simulink model "All_sensors_Ball_Plate_reduce_observer"  (R2018b)
settings: Solver=ode15s  StartTime=0.0  StopTime=100  RelTol=1e-3
undefined symbols (not defined in the file): A21, B2, Hb, K, K1, K2, K3, K4, X, Y, Z
libraries: sm_lib x16, nesl_utility x11, simulink x3
settings Model: Creator=Giorgio Cannata  LastModifiedBy=Francesca
settings SFSimCC: SimUseLocalCustomCode=off
settings RTWCC: RTWUseLocalCustomCode=off
settings CodeAppCC: StateflowObjectComments=on
settings SimscapeCC: SimscapeNormalizeSystem=off

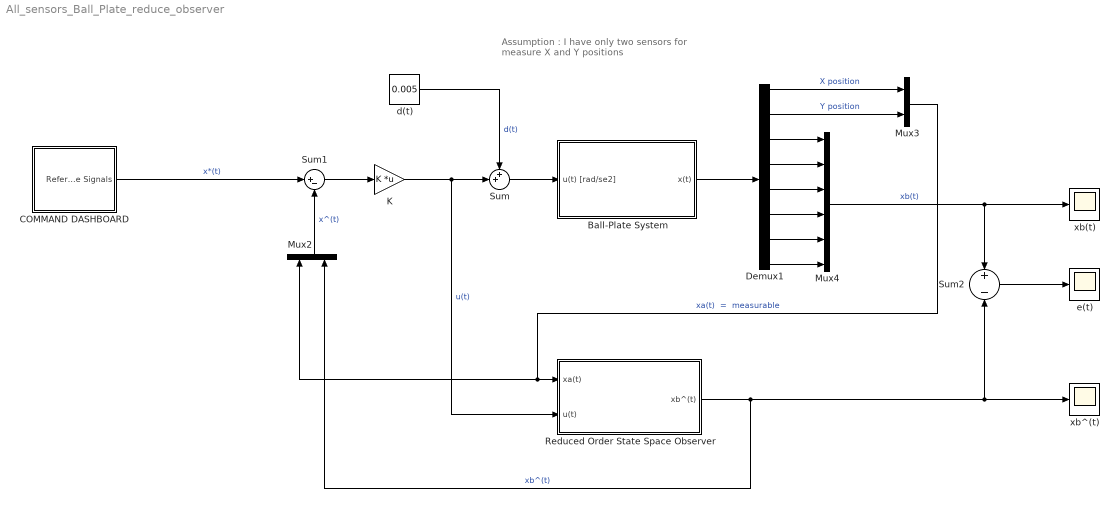
== system All_sensors_Ball_Plate_reduce_observer ==
  note: Assumption : I have only two sensors
      | for measure X and Y positions
  Ball-Plate System : Subsystem  mask{Px0=15, Py0=10, Vx0=0, Vy0=0, alfa0=0, beta0=0, w_alfa0=0, w_beta0=0}
      mask prompts: Px0 "Initial x position [mm]"; Py0 "Initial y position [mm]"; Vx0 "Initial x velocity [mm/sec]"; Vy0 "Initial y velocity [mm/sec]"; alfa0 "Initial alfa angle [deg]"; beta0 "Initial beta angle [deg]"; w_alfa0 "Initial w_alfa [deg/sec]"; w_beta0 "Initial w_beta [deg/sec]"
      mask init:
      | Px0 = Px0/1000;
      | Py0 = Py0/1000;
      | 
      | Vx0 = Vx0/1000;
      | Vy0 = Vy0/1000;
      | 
      | alfa0 = alfa0*pi/180;
      | beta0 = beta0*pi/180;
      | 
      | w_alfa0 = w_alfa0*pi/180;
      | w_beta0 = w_beta0*pi/180;
  COMMAND DASHBOARD : Subsystem
  Demux1 : Demux  Outputs=8
  K : Gain  Gain=K  Multiplication=Matrix(K*u)
  Mux2 : Mux  Inputs=2
  Mux3 : Mux  Inputs=2
  Mux4 : Mux  Inputs=6
  Reduced Order State Space Observer : Subsystem  mask{Hb=Hb, K1=K1, K2=K2, K3=K3, K4=K4}
      mask prompts: Hb "Matrix Hb"; K1 "K1=A22-Hb*A12"; K2 "K2=(A22-Hb*A12)*Hb"; K3 "K3=Hb*B1"; K4 "K4=Hb*A11"
  Sum : Sum  Inputs=++|
  Sum1 : Sum  Inputs=|+-
  Sum2 : Sum  Inputs=+|-
  d(t) : Constant  Value=0.005
  e(t) : Scope
  xb(t) : Scope
  xb^(t) : Scope
  wires:
  COMMAND DASHBOARD/1(Reference Signals) -> Sum1/1  "x*(t)"
  Sum2/1 -> e(t)/1
  K/1 -> Reduced Order State Space Observer/2(u(t)), Sum/2  "u(t)"
  Reduced Order State Space Observer/1(xb^(t)) -> Sum2/2, xb^(t)/1, Mux2/2  "xb^(t)"
  Sum1/1 -> K/1
  d(t)/1 -> Sum/1  "d(t)"
  Sum/1 -> Ball-Plate System/1(u(t) [rad/se2])
  Demux1/7 -> Mux4/5
  Demux1/2 -> Mux3/2  "Y position"
  Demux1/5 -> Mux4/3
  Mux4/1 -> xb(t)/1, Sum2/1  "xb(t)"
  Demux1/8 -> Mux4/6
  Demux1/6 -> Mux4/4
  Ball-Plate System/1(x(t)) -> Demux1/1
  Demux1/1 -> Mux3/1  "X position"
  Demux1/4 -> Mux4/2
  Mux3/1 -> Reduced Order State Space Observer/1(xa(t)), Mux2/1  "xa(t)  =  measurable"
  Demux1/3 -> Mux4/1
  Mux2/1 -> Sum1/2  "x^(t)"

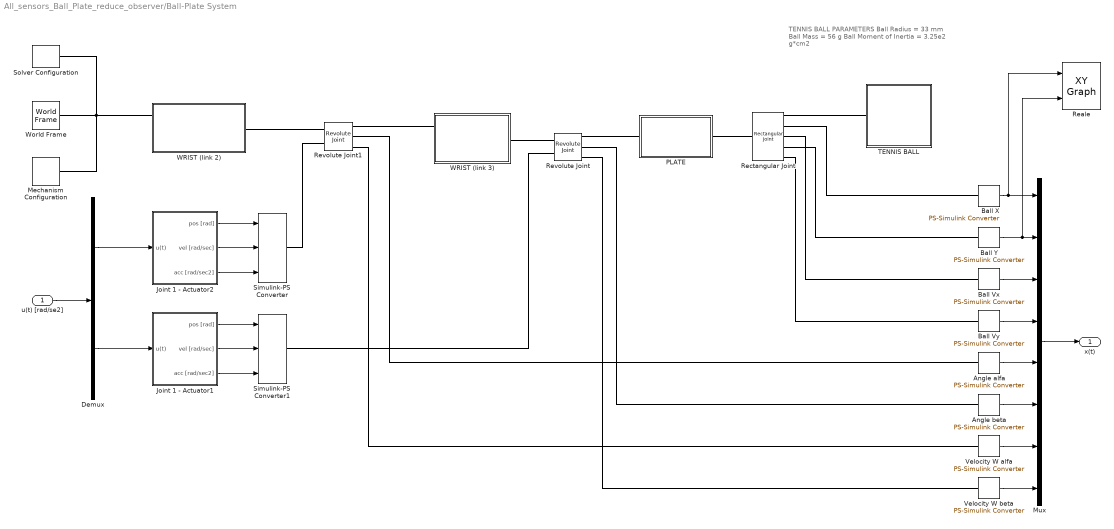
== system All_sensors_Ball_Plate_reduce_observer/Ball-Plate System ==
  note: TENNIS BALL PARAMETERS
      | Ball Radius = 33 mm
      | Ball Mass = 56 g
      | Ball Moment of Inertia = 3.25e2 g*cm2
  u(t) [rad/se2] : Inport
  Angle alfa : nesl_utility/PS-Simulink Converter  PhysicalDomain=network_engine_domain  SubClassName=ps_output  LeftPortType=input  RightPortType=output  PseudoPeriodic=off  Frequencies=[]  Unit=rad  AffineConversion=off
  Angle beta : nesl_utility/PS-Simulink Converter  PhysicalDomain=network_engine_domain  SubClassName=ps_output  LeftPortType=input  RightPortType=output  PseudoPeriodic=off  Frequencies=[]  Unit=rad  AffineConversion=off
  Ball Vx : nesl_utility/PS-Simulink Converter  PhysicalDomain=network_engine_domain  SubClassName=ps_output  LeftPortType=input  RightPortType=output  PseudoPeriodic=off  Frequencies=[]  Unit=m/s  AffineConversion=off
  Ball Vy : nesl_utility/PS-Simulink Converter  PhysicalDomain=network_engine_domain  SubClassName=ps_output  LeftPortType=input  RightPortType=output  PseudoPeriodic=off  Frequencies=[]  Unit=m/s  AffineConversion=off
  Ball X : nesl_utility/PS-Simulink Converter  PhysicalDomain=network_engine_domain  SubClassName=ps_output  LeftPortType=input  RightPortType=output  PseudoPeriodic=off  Frequencies=[]  Unit=m  AffineConversion=off
  Ball Y : nesl_utility/PS-Simulink Converter  PhysicalDomain=network_engine_domain  SubClassName=ps_output  LeftPortType=input  RightPortType=output  PseudoPeriodic=off  Frequencies=[]  Unit=m  AffineConversion=off
  Demux : Demux  Outputs=2
  Joint 1 - Actuator1 : Subsystem  mask{Kp=0, Kv=0, G=1, p0=0, v0=0}
      mask prompts: G "Gain"; p0 "Initial Position [deg]"; v0 "Initial Velocity [deg/sec]"
      mask init:
      | p0 = p0 * pi/180
      | v0 = v0 * pi/180
  Joint 1 - Actuator2 : Subsystem  mask{Kp=0, Kv=0, G=1, p0=0, v0=0}
      mask prompts: G "Gain"; p0 "Initial Position [deg]"; v0 "Initial Velocity [deg/sec]"
      mask init:
      | p0 = p0 * pi/180
      | v0 = v0 * pi/180
  Mechanism Configuration : sm_lib/Utilities/Mechanism Configuration  UniformGravity=Constant  GravityVector=[0 0 -9.80665]  GravityUnits=m/s^2  LinearizationDelta=0.001
  Mux : Mux  Inputs=8
  PLATE : Subsystem  mask{L=400, W=400, T=10, Offset=100}
      mask prompts: L "Plate length [mm]"; W "Plate width [mm]"; T "Plate thickness [mm]"; Offset "Offset [mm]"
  Reale : simulink/Sinks/XY Graph  xmin=-1  xmax=1  ymin=-1  ymax=1  st=-1
  Rectangular Joint : sm_lib/Joints/Rectangular Joint  SenseConstraintForce=off  SenseConstraintForceX=off  SenseConstraintForceY=off  SenseConstraintForceZ=off  SenseConstraintTorque=off  SenseConstraintTorqueX=off  SenseConstraintTorqueY=off  SenseConstraintTorqueZ=off  SenseTotalForce=off  SenseTotalForceX=off  SenseTotalForceY=off  SenseTotalForceZ=off  SenseTotalTorque=off  SenseTotalTorqueX=off  SenseTotalTorqueY=off  SenseTotalTorqueZ=off  CompositeWrenchDir=FollowerOnBase  CompositeWrenchFrame=BaseFrame  PxEquilibriumPosition=0  PxEquilibriumPositionUnits=m  PxSpringStiffness=0  PxSpringStiffnessUnits=N/m  PxDampingCoefficient=0  PxDampingCoefficientUnits=N/(m/s)  PxTorqueActuationMode=NoTorque  PxMotionActuationMode=ComputedMotion  PxSensePosition=on  PxSenseVelocity=on  PxSenseAcceleration=off  PxSenseTorqueForce=off  PxPositionTargetSpecify=on  PxPositionTargetPriority=High  PxPositionTargetValue=Px0  PxPositionTargetValueUnits=m  PxVelocityTargetSpecify=on  PxVelocityTargetPriority=High  PxVelocityTargetValue=Vx0  PxVelocityTargetValueUnits=m/s  PyEquilibriumPosition=0  PyEquilibriumPositionUnits=m  PySpringStiffness=0  PySpringStiffnessUnits=N/m  PyDampingCoefficient=0  PyDampingCoefficientUnits=N/(m/s)  PyTorqueActuationMode=NoTorque  PyMotionActuationMode=ComputedMotion  PySensePosition=on  PySenseVelocity=on  PySenseAcceleration=off  PySenseTorqueForce=off  PyPositionTargetSpecify=on  PyPositionTargetPriority=High  PyPositionTargetValue=Py0  PyPositionTargetValueUnits=m  PyVelocityTargetSpecify=on  PyVelocityTargetPriority=High  PyVelocityTargetValue=Vy0  PyVelocityTargetValueUnits=m/s
      settings: SourceProductName=Simscape Multibody
  Revolute Joint : sm_lib/Joints/Revolute Joint  SenseConstraintForce=off  SenseConstraintForceX=off  SenseConstraintForceY=off  SenseConstraintForceZ=off  SenseConstraintTorque=off  SenseConstraintTorqueX=off  SenseConstraintTorqueY=off  SenseConstraintTorqueZ=off  SenseTotalForce=off  SenseTotalForceX=off  SenseTotalForceY=off  SenseTotalForceZ=off  SenseTotalTorque=off  SenseTotalTorqueX=off  SenseTotalTorqueY=off  SenseTotalTorqueZ=off  CompositeWrenchDir=FollowerOnBase  CompositeWrenchFrame=BaseFrame  EquilibriumPosition=0  EquilibriumPositionUnits=deg  SpringStiffness=0  SpringStiffnessUnits=N*m/deg  DampingCoefficient=0  DampingCoefficientUnits=N*m/(deg/s)  TorqueActuationMode=ComputedTorque  MotionActuationMode=InputMotion  SensePosition=on  SenseVelocity=on  SenseAcceleration=off  SenseTorqueForce=off  PositionTargetSpecify=off  PositionTargetPriority=High  PositionTargetValue=0  PositionTargetValueUnits=deg  VelocityTargetSpecify=off  VelocityTargetPriority=High  VelocityTargetValue=0  VelocityTargetValueUnits=deg/s
  Revolute Joint1 : sm_lib/Joints/Revolute Joint  SenseConstraintForce=off  SenseConstraintForceX=off  SenseConstraintForceY=off  SenseConstraintForceZ=off  SenseConstraintTorque=off  SenseConstraintTorqueX=off  SenseConstraintTorqueY=off  SenseConstraintTorqueZ=off  SenseTotalForce=off  SenseTotalForceX=off  SenseTotalForceY=off  SenseTotalForceZ=off  SenseTotalTorque=off  SenseTotalTorqueX=off  SenseTotalTorqueY=off  SenseTotalTorqueZ=off  CompositeWrenchDir=FollowerOnBase  CompositeWrenchFrame=BaseFrame  EquilibriumPosition=0  EquilibriumPositionUnits=deg  SpringStiffness=0  SpringStiffnessUnits=N*m/deg  DampingCoefficient=0  DampingCoefficientUnits=N*m/(deg/s)  TorqueActuationMode=ComputedTorque  MotionActuationMode=InputMotion  SensePosition=on  SenseVelocity=on  SenseAcceleration=off  SenseTorqueForce=off  PositionTargetSpecify=off  PositionTargetPriority=High  PositionTargetValue=0  PositionTargetValueUnits=deg  VelocityTargetSpecify=off  VelocityTargetPriority=High  VelocityTargetValue=0  VelocityTargetValueUnits=deg/s
  Simulink-PS Converter : nesl_utility/Simulink-PS Converter  PhysicalDomain=network_engine_domain  SubClassName=ps_input  LeftPortType=input  RightPortType=output  PseudoPeriodic=off  Frequencies=[]  NoiseDistribution=none  NoiseParameters=[]  Unit=1  AffineConversion=off  FilteringAndDerivatives=provide  SimscapeFilterOrder=1  InputFilterTimeConstant=0.001  UdotUserProvided=2
  Simulink-PS Converter1 : nesl_utility/Simulink-PS Converter  PhysicalDomain=network_engine_domain  SubClassName=ps_input  LeftPortType=input  RightPortType=output  PseudoPeriodic=off  Frequencies=[]  NoiseDistribution=none  NoiseParameters=[]  Unit=1  AffineConversion=off  FilteringAndDerivatives=provide  SimscapeFilterOrder=1  InputFilterTimeConstant=0.001  UdotUserProvided=2
  Solver Configuration : nesl_utility/Solver Configuration  PhysicalDomain=network_engine_domain  SubClassName=solver  LeftPortType=input  RightPortType=generic  Tones=[]  Harmonics=[]  SimulateNoise=off  Profile=off  UseLocalSampling=off  EnableSwitchedLinearOptims=on  FrequencyDomain=off  UseCCode=off  RelTol=0.001  AbsTol=1e-06  MinStep=1e-09  ToWorkspace=off  RevertToSquareIcSolve=off  NumHomotopyIterations=100  PhasorMode=off  PhasorModeNumHarmonics=1  DoDC=off  ResidualTolerance=1e-09  UseLocalSolver=off  LocalSolverChoice=NE_BACKWARD_EULER_ADVANCER  LocalSolverSampleTime=0.0005  DoFixedCost=off  MaxNonlinIter=3  MaxModeIter=2  LinearAlgebra=Sparse  EquationFormulation=NE_TIME_EF  DelaysMemoryBudget=1024  AutomaticFiltering=on  FilteringTimeConstant=0.001  PartitionStorageMethod=AS_NEEDED  PartitionMemoryBudget=1024
  TENNIS BALL : Subsystem  mask{rb=33, mb=56, Ib=3.25e2}
      mask prompts: rb "Ball radius [mm]"; mb "Ball mass [g]"; Ib "Ball momentum of inertia [g cm2]"
      mask init:
      | Ib = 10^4 * Ib; % Trasnfor to [g*mm]
      | m = mb + Ib/rb^2; % Equivalent inertia - as a sliding object
      mask Display: image('TennisBall.png');
  Velocity W alfa : nesl_utility/PS-Simulink Converter  PhysicalDomain=network_engine_domain  SubClassName=ps_output  LeftPortType=input  RightPortType=output  PseudoPeriodic=off  Frequencies=[]  Unit=rad/s  AffineConversion=off
  Velocity W beta : nesl_utility/PS-Simulink Converter  PhysicalDomain=network_engine_domain  SubClassName=ps_output  LeftPortType=input  RightPortType=output  PseudoPeriodic=off  Frequencies=[]  Unit=rad/s  AffineConversion=off
  WRIST (link 2) : Subsystem  mask{L=150, R=80}
      mask prompts: L "Length [mm]"; R "Radius [mm]"
  WRIST (link 3) : Subsystem  mask{L=300, R=65}
      mask prompts: L "Link length [mm]"; R "Link radius [mm]"
  World Frame : sm_lib/Frames and Transforms/World Frame
  x(t) : Outport
  wires:
  Angle alfa/1 -> Mux/5
  Ball Vy/1 -> Mux/4
  Angle beta/1 -> Mux/6
  Ball Vx/1 -> Mux/3
  Ball Y/1 -> Reale/2, Mux/2
  Velocity W alfa/1 -> Mux/7
  Ball X/1 -> Mux/1, Reale/1
  Velocity W beta/1 -> Mux/8
  u(t) [rad/se2]/1 -> Demux/1
  Mux/1 -> x(t)/1
  Demux/1 -> Joint 1 - Actuator2/1(u(t))
  Joint 1 - Actuator2/1(pos [rad]) -> Simulink-PS Converter/1
  Joint 1 - Actuator2/2(vel [rad/sec]) -> Simulink-PS Converter/2
  Joint 1 - Actuator2/3(acc [rad/sec2]) -> Simulink-PS Converter/3
  Joint 1 - Actuator1/1(pos [rad]) -> Simulink-PS Converter1/1
  Joint 1 - Actuator1/2(vel [rad/sec]) -> Simulink-PS Converter1/2
  Joint 1 - Actuator1/3(acc [rad/sec2]) -> Simulink-PS Converter1/3
  Demux/2 -> Joint 1 - Actuator1/1(u(t))
  connections:
  WRIST (link 3)/RConn1 -- Revolute Joint/LConn1
  Revolute Joint1/LConn1 -- WRIST (link 2)/RConn1
  Revolute Joint/RConn1 -- PLATE/LConn1
  PLATE/RConn1 -- Rectangular Joint/LConn1
  TENNIS BALL/LConn1 -- Rectangular Joint/RConn1
  Ball X/LConn1 -- Rectangular Joint/RConn2
  Revolute Joint1/RConn1 -- WRIST (link 3)/LConn1
  Solver Configuration/RConn1 -- WRIST (link 2)/LConn1 -- Mechanism Configuration/RConn1 -- World Frame/RConn1
  Rectangular Joint/RConn4 -- Ball Y/LConn1
  Rectangular Joint/RConn3 -- Ball Vx/LConn1
  Rectangular Joint/RConn5 -- Ball Vy/LConn1
  Revolute Joint/RConn2 -- Angle beta/LConn1
  Revolute Joint1/RConn2 -- Angle alfa/LConn1
  Revolute Joint1/RConn3 -- Velocity W alfa/LConn1
  Revolute Joint/RConn3 -- Velocity W beta/LConn1
  Simulink-PS Converter/RConn1 -- Revolute Joint1/LConn2
  Simulink-PS Converter1/RConn1 -- Revolute Joint/LConn2

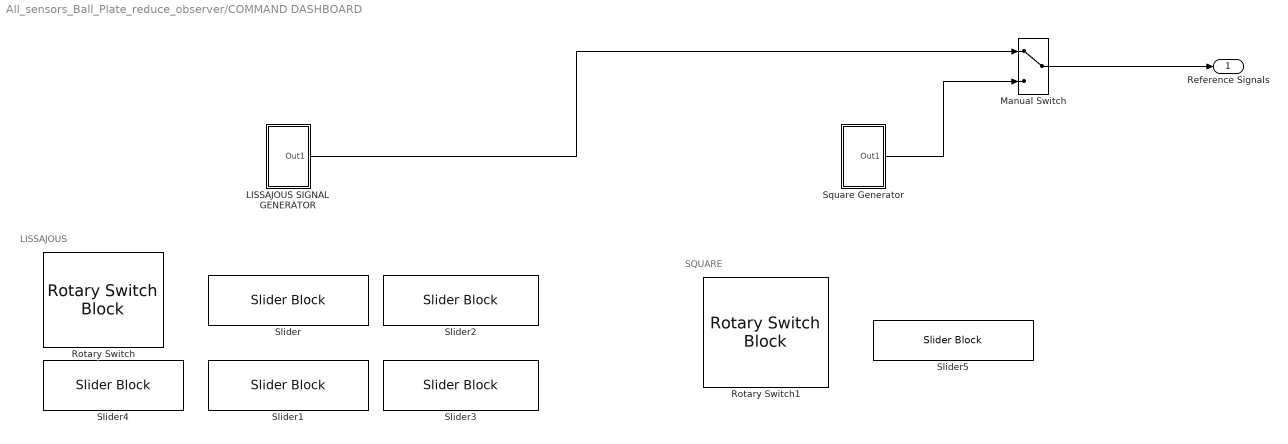
== system All_sensors_Ball_Plate_reduce_observer/COMMAND DASHBOARD ==
  note: SQUARE
  note: LISSAJOUS
  LISSAJOUS SIGNAL GENERATOR : Subsystem
  Manual Switch : ManualSwitch
  Rotary Switch : RotarySwitchBlock  WebBlockId=121
      settings: Values={{'X-Y', 'L (1-1)', 'L (1-2)', 'L (3-2)', 'L (3-4)', 'L (5-4)'}, [0 1 2 3 4 5]}
  Rotary Switch1 : RotarySwitchBlock  WebBlockId=120
      settings: Values={{'Low', 'Low-Med', 'Med-High', 'High', 'Very-High'}, [3 5 7 9 11]}
  Slider : SliderBlock  WebBlockId=119  ScaleMax=0.20000000000000001
  Slider1 : SliderBlock  WebBlockId=118  ScaleMax=0.20000000000000001
  Slider2 : SliderBlock  WebBlockId=117  ScaleMin=-0.20000000000000001  ScaleMax=0.20000000000000001
  Slider3 : SliderBlock  WebBlockId=115  ScaleMin=-0.20000000000000001  ScaleMax=0.20000000000000001
  Slider4 : SliderBlock  WebBlockId=116  ScaleMax=1
  Slider5 : SliderBlock  WebBlockId=114  ScaleMax=2
  Square Generator : Subsystem
  Reference Signals : Outport
  wires:
  Square Generator/1(Out1) -> Manual Switch/2
  Manual Switch/1 -> Reference Signals/1
  LISSAJOUS SIGNAL GENERATOR/1(Out1) -> Manual Switch/1

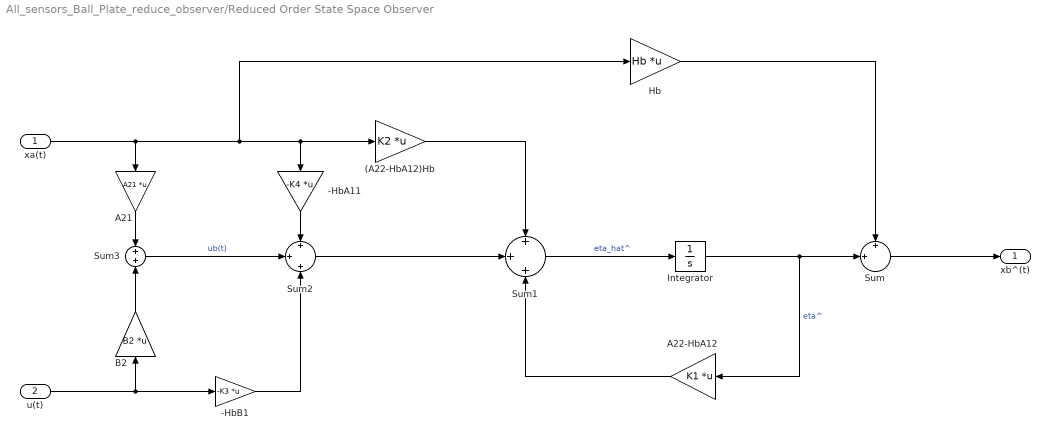
== system All_sensors_Ball_Plate_reduce_observer/Reduced Order State Space Observer ==
  xa(t) : Inport
  u(t) : Inport  Port=2
  (A22-HbA12)Hb : Gain  Gain=K2  Multiplication=Matrix(K*u)
  -HbA11 : Gain  Gain=-K4  Multiplication=Matrix(K*u)
  -HbB1 : Gain  Gain=-K3  Multiplication=Matrix(K*u)
  A21 : Gain  Gain=A21  Multiplication=Matrix(K*u)
  A22-HbA12 : Gain  Gain=K1  Multiplication=Matrix(K*u)
  B2 : Gain  Gain=B2  Multiplication=Matrix(K*u)
  Hb : Gain  Gain=Hb  Multiplication=Matrix(K*u)
  Integrator : Integrator
  Sum : Sum  Inputs=+|+||
  Sum1 : Sum  Inputs=+|+|+
  Sum2 : Sum  Inputs=+|+|+
  Sum3 : Sum  Inputs=+|+
  xb^(t) : Outport
  wires:
  Hb/1 -> Sum/1
  A21/1 -> Sum3/1
  (A22-HbA12)Hb/1 -> Sum1/1
  B2/1 -> Sum3/2
  A22-HbA12/1 -> Sum1/3
  u(t)/1 -> -HbB1/1, B2/1
  Sum1/1 -> Integrator/1  "eta_hat^"
  -HbA11/1 -> Sum2/1
  Sum2/1 -> Sum1/2
  Sum/1 -> xb^(t)/1
  Integrator/1 -> Sum/2, A22-HbA12/1  "eta^"
  xa(t)/1 -> Hb/1, -HbA11/1, (A22-HbA12)Hb/1, A21/1
  Sum3/1 -> Sum2/2  "ub(t)"
  -HbB1/1 -> Sum2/3

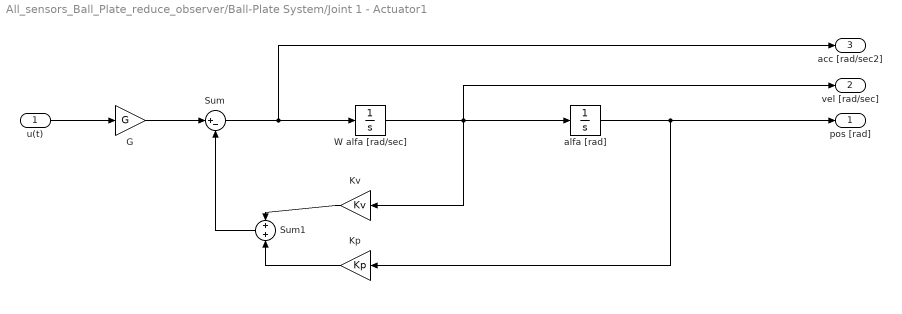
== system All_sensors_Ball_Plate_reduce_observer/Ball-Plate System/Joint 1 - Actuator1 ==
  u(t) : Inport
  G : Gain  Gain=G
  Kp : Gain  Gain=Kp
  Kv : Gain  Gain=Kv
  Sum : Sum  Inputs=|+-
  Sum1 : Sum  Inputs=+|+
  W alfa [rad/sec] : Integrator  InitialCondition=v0
  alfa [rad] : Integrator  InitialCondition=p0
  pos [rad] : Outport
  vel [rad/sec] : Outport  Port=2
  acc [rad/sec2] : Outport  Port=3
  wires:
  Sum1/1 -> Sum/2
  Kp/1 -> Sum1/2
  Kv/1 -> Sum1/1
  G/1 -> Sum/1
  Sum/1 -> W alfa [rad/sec]/1, acc [rad/sec2]/1
  alfa [rad]/1 -> pos [rad]/1, Kp/1
  W alfa [rad/sec]/1 -> alfa [rad]/1, vel [rad/sec]/1, Kv/1
  u(t)/1 -> G/1

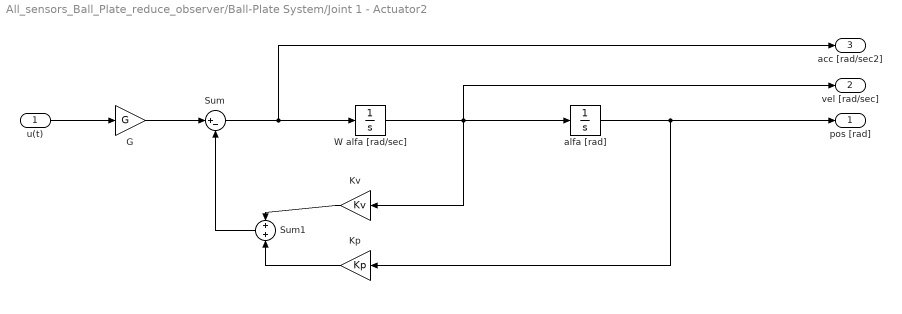
== system All_sensors_Ball_Plate_reduce_observer/Ball-Plate System/Joint 1 - Actuator2 ==
  u(t) : Inport
  G : Gain  Gain=G
  Kp : Gain  Gain=Kp
  Kv : Gain  Gain=Kv
  Sum : Sum  Inputs=|+-
  Sum1 : Sum  Inputs=+|+
  W alfa [rad/sec] : Integrator  InitialCondition=v0
  alfa [rad] : Integrator  InitialCondition=p0
  pos [rad] : Outport
  vel [rad/sec] : Outport  Port=2
  acc [rad/sec2] : Outport  Port=3
  wires:
  u(t)/1 -> G/1
  W alfa [rad/sec]/1 -> Kv/1, vel [rad/sec]/1, alfa [rad]/1
  alfa [rad]/1 -> Kp/1, pos [rad]/1
  Sum/1 -> acc [rad/sec2]/1, W alfa [rad/sec]/1
  G/1 -> Sum/1
  Kv/1 -> Sum1/1
  Kp/1 -> Sum1/2
  Sum1/1 -> Sum/2

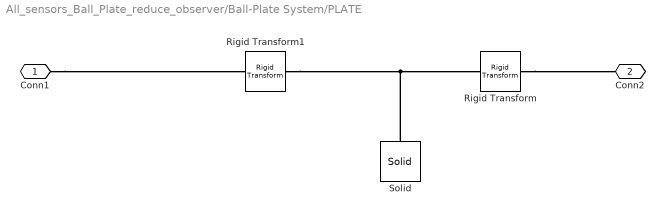
== system All_sensors_Ball_Plate_reduce_observer/Ball-Plate System/PLATE ==
  Rigid Transform : sm_lib/Frames and Transforms/Rigid Transform  TranslationMethod=StandardAxis  TranslationStandardOffset=T/2  TranslationLengthUnit=mm  TranslationStandardAxis=+Z  TranslationCartesianOffset=[0 0 0]  TranslationROffset=0  TranslationROffsetUnits=m  TranslationZOffset=0  TranslationZOffsetUnits=m  TranslationThetaOffset=0  TranslationThetaOffsetUnits=deg  RotationMethod=None  RotationAngleUnits=deg  RotationStandardAxis=+Z  RotationAngle=0.0  RotationArbitraryAxis=[0 0 1]  FollAlignAxisA=+X  BaseAlignAxisA=+Y  FollAlignAxisB=+Y  BaseAlignAxisB=+Z  RotationSequenceAxes=FollowerAxes  RotationSequence=XYX  RotationSequenceAngles=[0 0 0]  RotationSequenceAnglesUnits=deg  RotationMatrix=[1 0 0; 0 1 0; 0 0 1]
  Rigid Transform1 : sm_lib/Frames and Transforms/Rigid Transform  TranslationMethod=StandardAxis  TranslationStandardOffset=Offset-T/2  TranslationLengthUnit=mm  TranslationStandardAxis=-Z  TranslationCartesianOffset=[0 0 0]  TranslationROffset=0  TranslationROffsetUnits=m  TranslationZOffset=0  TranslationZOffsetUnits=m  TranslationThetaOffset=0  TranslationThetaOffsetUnits=deg  RotationMethod=StandardAxis  RotationAngleUnits=deg  RotationStandardAxis=-X  RotationAngle=90.0  RotationArbitraryAxis=[1 0 0]  FollAlignAxisA=+X  BaseAlignAxisA=+Y  FollAlignAxisB=+Y  BaseAlignAxisB=+Z  RotationSequenceAxes=FollowerAxes  RotationSequence=XYX  RotationSequenceAngles=[0 0 0]  RotationSequenceAnglesUnits=deg  RotationMatrix=[1 0 0; 0 1 0; 0 0 1]
  Solid : sm_lib/Body Elements/Solid  InertiaType=CalculateFromGeometry  Mass=1  MassUnits=kg  CenterOfMass=[0 0 0]  CenterOfMassUnits=m  MomentsOfInertia=[1 1 1]  MomentsOfInertiaUnits=kg*m^2  ProductsOfInertia=[0 0 0]  ProductsOfInertiaUnits=kg*m^2  BasedOnType=Density  Density=0  DensityUnits=kg/(m^3)  DoExposeReferenceFrame=on  SerializedFrames=<Frames/>  GraphicType=FromGeometry  MarkerShape=Sphere  MarkerSize=10  GraphicVisPropType=SimpleVisualProperties  GraphicDiffuseColor=[0.65 0.65 0.65]  GraphicSpecularColor=[0.5 0.5 0.5 1.0]  GraphicAmbientColor=[0.15 0.15 0.15 1.0]  GraphicEmissiveColor=[0.0 0.0 0.0 1.0]  GraphicShininess=75  GraphicOpacity=1.0  GeometryShape=Brick  RectangleSize=[1 1]  RectangleSizeUnits=m  BrickDimensions=[L W T]  BrickDimensionUnits=mm  CylinderRadius=1  CylinderRadiusUnits=m  CylinderLength=1  CylinderLengthUnits=m  SphereRadius=1  SphereRadiusUnits=m  EllipsoidRadii=[1 1 1]  EllipsoidRadiiUnits=m  ExtrusionCrossSection=[1 1; -1 1; -1 -1; 1 -1]  ExtrusionCrossSectionUnits=m  ExtrusionLength=1  ExtrusionLengthUnits=m  PolygonNumSides=3  PolygonOuterRadius=1  PolygonOuterRadiusUnits=m  ExtGeomFileType=STEP  ExtGeomFileUnits=m  RevolutionCrossSection=[1 1; 1 -1; 2 -1; 2 1]  RevolutionCrossSectionUnits=m  RevolutionExtent=Full  RevolutionAngle=180  RevolutionAngleUnits=deg
  Conn1 : PMIOPort  Side=Left
  Conn2 : PMIOPort  Port=2  Side=Right
  connections:
  Rigid Transform/RConn1 -- Conn2/RConn1
  Conn1/RConn1 -- Rigid Transform1/RConn1
  Rigid Transform1/LConn1 -- Solid/RConn1 -- Rigid Transform/LConn1

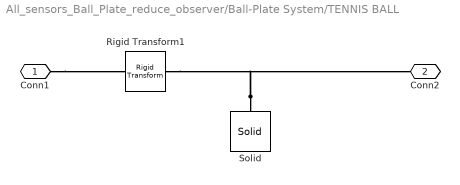
== system All_sensors_Ball_Plate_reduce_observer/Ball-Plate System/TENNIS BALL ==
  Rigid Transform1 : sm_lib/Frames and Transforms/Rigid Transform  TranslationMethod=StandardAxis  TranslationStandardOffset=rb  TranslationLengthUnit=mm  TranslationStandardAxis=-Z  TranslationCartesianOffset=[0 0 0]  TranslationROffset=0  TranslationROffsetUnits=m  TranslationZOffset=0  TranslationZOffsetUnits=m  TranslationThetaOffset=0  TranslationThetaOffsetUnits=deg  RotationMethod=None  RotationAngleUnits=deg  RotationStandardAxis=+Z  RotationAngle=0.0  RotationArbitraryAxis=[0 0 1]  FollAlignAxisA=+X  BaseAlignAxisA=+Y  FollAlignAxisB=+Y  BaseAlignAxisB=+Z  RotationSequenceAxes=FollowerAxes  RotationSequence=XYX  RotationSequenceAngles=[0 0 0]  RotationSequenceAnglesUnits=deg  RotationMatrix=[1 0 0; 0 1 0; 0 0 1]
  Solid : sm_lib/Body Elements/Solid  InertiaType=Custom  Mass=m  MassUnits=g  CenterOfMass=[0 0 0]  CenterOfMassUnits=mm  MomentsOfInertia=[1 1 1]*0  MomentsOfInertiaUnits=g*cm^2  ProductsOfInertia=[0 0 0]  ProductsOfInertiaUnits=kg*m^2  BasedOnType=Density  Density=1000  DensityUnits=kg/(m^3)  DoExposeReferenceFrame=on  SerializedFrames=<Frames/>  GraphicType=FromGeometry  MarkerShape=Sphere  MarkerSize=10  GraphicVisPropType=AdvancedVisualProperties  GraphicDiffuseColor=[1 1 0]  GraphicSpecularColor=[1 1 0 1]  GraphicAmbientColor=[0.15 0.15 0.15 1.0]  GraphicEmissiveColor=[0.1 0.1 0.0 1.0]  GraphicShininess=10  GraphicOpacity=1.0  GeometryShape=Sphere  RectangleSize=[1 1]  RectangleSizeUnits=m  BrickDimensions=[1 1 1]  BrickDimensionUnits=m  CylinderRadius=1  CylinderRadiusUnits=m  CylinderLength=1  CylinderLengthUnits=m  SphereRadius=rb  SphereRadiusUnits=mm  EllipsoidRadii=[1 1 1]  EllipsoidRadiiUnits=m  ExtrusionCrossSection=[1 1; -1 1; -1 -1; 1 -1]  ExtrusionCrossSectionUnits=m  ExtrusionLength=1  ExtrusionLengthUnits=m  PolygonNumSides=3  PolygonOuterRadius=1  PolygonOuterRadiusUnits=m  ExtGeomFileType=STEP  ExtGeomFileUnits=m  RevolutionCrossSection=[1 1; 1 -1; 2 -1; 2 1]  RevolutionCrossSectionUnits=m  RevolutionExtent=Full  RevolutionAngle=180  RevolutionAngleUnits=deg
  Conn1 : PMIOPort  Side=Left
  Conn2 : PMIOPort  Port=2  Side=Right
  connections:
  Conn1/RConn1 -- Rigid Transform1/RConn1
  Solid/RConn1 -- Rigid Transform1/LConn1 -- Conn2/RConn1

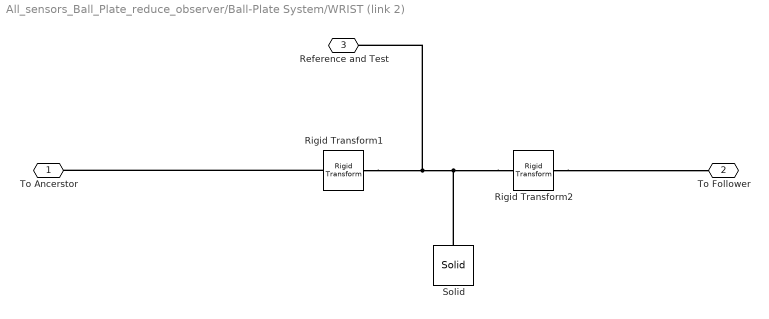
== system All_sensors_Ball_Plate_reduce_observer/Ball-Plate System/WRIST (link 2) ==
  Rigid Transform1 : sm_lib/Frames and Transforms/Rigid Transform  TranslationMethod=None  TranslationStandardOffset=L/2  TranslationLengthUnit=mm  TranslationStandardAxis=-Z  TranslationCartesianOffset=[0 0 0]  TranslationROffset=0  TranslationROffsetUnits=m  TranslationZOffset=0  TranslationZOffsetUnits=m  TranslationThetaOffset=0  TranslationThetaOffsetUnits=deg  RotationMethod=StandardAxis  RotationAngleUnits=deg  RotationStandardAxis=+Y  RotationAngle=-90.0  RotationArbitraryAxis=[1 0 0]  FollAlignAxisA=+X  BaseAlignAxisA=+Y  FollAlignAxisB=+Y  BaseAlignAxisB=+Z  RotationSequenceAxes=FollowerAxes  RotationSequence=XYX  RotationSequenceAngles=[0 0 0]  RotationSequenceAnglesUnits=deg  RotationMatrix=[1 0 0; 0 1 0; 0 0 1]
  Rigid Transform2 : sm_lib/Frames and Transforms/Rigid Transform  TranslationMethod=None  TranslationStandardOffset=L/2  TranslationLengthUnit=mm  TranslationStandardAxis=+Z  TranslationCartesianOffset=[0 0 0]  TranslationROffset=0  TranslationROffsetUnits=m  TranslationZOffset=0  TranslationZOffsetUnits=m  TranslationThetaOffset=0  TranslationThetaOffsetUnits=deg  RotationMethod=None  RotationAngleUnits=deg  RotationStandardAxis=+Z  RotationAngle=-90.0  RotationArbitraryAxis=[1 0 0]  FollAlignAxisA=+X  BaseAlignAxisA=+Y  FollAlignAxisB=+Y  BaseAlignAxisB=+Z  RotationSequenceAxes=FollowerAxes  RotationSequence=XYX  RotationSequenceAngles=[0 0 0]  RotationSequenceAnglesUnits=deg  RotationMatrix=[1 0 0; 0 1 0; 0 0 1]
  Solid : sm_lib/Body Elements/Solid  InertiaType=CalculateFromGeometry  Mass=1  MassUnits=kg  CenterOfMass=[0 0 0]  CenterOfMassUnits=m  MomentsOfInertia=[1 1 1]  MomentsOfInertiaUnits=kg*m^2  ProductsOfInertia=[0 0 0]  ProductsOfInertiaUnits=kg*m^2  BasedOnType=Density  Density=0  DensityUnits=kg/(m^3)  DoExposeReferenceFrame=on  SerializedFrames=<Frames/>  GraphicType=FromGeometry  MarkerShape=Sphere  MarkerSize=10  GraphicVisPropType=SimpleVisualProperties  GraphicDiffuseColor=[0.65 00.15 0.35]  GraphicSpecularColor=[0.5 0.5 0.5 1.0]  GraphicAmbientColor=[0.15 0.15 0.15 1.0]  GraphicEmissiveColor=[0.0 0.0 0.0 1.0]  GraphicShininess=75  GraphicOpacity=1.0  GeometryShape=Cylinder  RectangleSize=[1 1]  RectangleSizeUnits=m  BrickDimensions=[1 1 1]  BrickDimensionUnits=m  CylinderRadius=R  CylinderRadiusUnits=mm  CylinderLength=L  CylinderLengthUnits=mm  SphereRadius=1  SphereRadiusUnits=m  EllipsoidRadii=[1 1 1]  EllipsoidRadiiUnits=m  ExtrusionCrossSection=[1 1; -1 1; -1 -1; 1 -1]  ExtrusionCrossSectionUnits=m  ExtrusionLength=1  ExtrusionLengthUnits=m  PolygonNumSides=3  PolygonOuterRadius=1  PolygonOuterRadiusUnits=m  ExtGeomFileType=STEP  ExtGeomFileUnits=m  RevolutionCrossSection=[1 1; 1 -1; 2 -1; 2 1]  RevolutionCrossSectionUnits=m  RevolutionExtent=Full  RevolutionAngle=180  RevolutionAngleUnits=deg
  To Ancerstor : PMIOPort  Side=Left
  To Follower : PMIOPort  Port=2  Side=Right
  Reference and Test : PMIOPort  Port=3  Side=Left
  connections:
  Rigid Transform2/LConn1 -- Reference and Test/RConn1 -- Rigid Transform1/LConn1 -- Solid/RConn1
  Rigid Transform1/RConn1 -- To Ancerstor/RConn1
  Rigid Transform2/RConn1 -- To Follower/RConn1

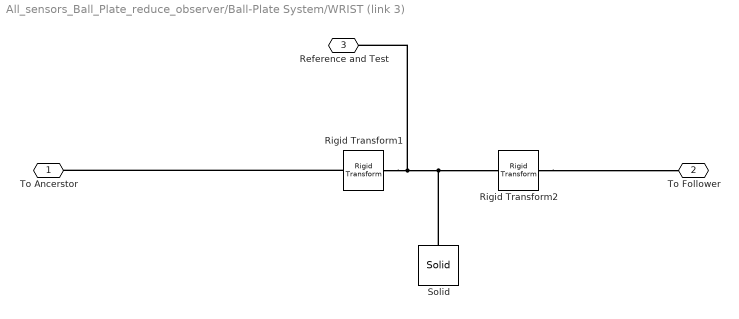
== system All_sensors_Ball_Plate_reduce_observer/Ball-Plate System/WRIST (link 3) ==
  Rigid Transform1 : sm_lib/Frames and Transforms/Rigid Transform  TranslationMethod=StandardAxis  TranslationStandardOffset=L/2  TranslationLengthUnit=mm  TranslationStandardAxis=-Z  TranslationCartesianOffset=[0 0 0]  TranslationROffset=0  TranslationROffsetUnits=m  TranslationZOffset=0  TranslationZOffsetUnits=m  TranslationThetaOffset=0  TranslationThetaOffsetUnits=deg  RotationMethod=StandardAxis  RotationAngleUnits=deg  RotationStandardAxis=+X  RotationAngle=90.0  RotationArbitraryAxis=[1 0 0]  FollAlignAxisA=+X  BaseAlignAxisA=+Y  FollAlignAxisB=+Y  BaseAlignAxisB=+Z  RotationSequenceAxes=FollowerAxes  RotationSequence=XYX  RotationSequenceAngles=[0 0 0]  RotationSequenceAnglesUnits=deg  RotationMatrix=[1 0 0; 0 1 0; 0 0 1]
  Rigid Transform2 : sm_lib/Frames and Transforms/Rigid Transform  TranslationMethod=StandardAxis  TranslationStandardOffset=L/2  TranslationLengthUnit=mm  TranslationStandardAxis=+Z  TranslationCartesianOffset=[0 0 0]  TranslationROffset=0  TranslationROffsetUnits=m  TranslationZOffset=0  TranslationZOffsetUnits=m  TranslationThetaOffset=0  TranslationThetaOffsetUnits=deg  RotationMethod=StandardAxis  RotationAngleUnits=deg  RotationStandardAxis=+Z  RotationAngle=-90.0  RotationArbitraryAxis=[1 0 0]  FollAlignAxisA=+X  BaseAlignAxisA=+Y  FollAlignAxisB=+Y  BaseAlignAxisB=+Z  RotationSequenceAxes=FollowerAxes  RotationSequence=XYX  RotationSequenceAngles=[0 0 0]  RotationSequenceAnglesUnits=deg  RotationMatrix=[1 0 0; 0 1 0; 0 0 1]
  Solid : sm_lib/Body Elements/Solid  InertiaType=CalculateFromGeometry  Mass=1  MassUnits=kg  CenterOfMass=[0 0 0]  CenterOfMassUnits=m  MomentsOfInertia=[1 1 1]  MomentsOfInertiaUnits=kg*m^2  ProductsOfInertia=[0 0 0]  ProductsOfInertiaUnits=kg*m^2  BasedOnType=Density  Density=0  DensityUnits=kg/(m^3)  DoExposeReferenceFrame=on  SerializedFrames=<Frames/>  GraphicType=FromGeometry  MarkerShape=Sphere  MarkerSize=10  GraphicVisPropType=SimpleVisualProperties  GraphicDiffuseColor=[0.65 0 0]  GraphicSpecularColor=[0.5 0.5 0.5 1.0]  GraphicAmbientColor=[0.15 0.15 0.15 1.0]  GraphicEmissiveColor=[0.0 0.0 0.0 1.0]  GraphicShininess=75  GraphicOpacity=1.0  GeometryShape=Cylinder  RectangleSize=[1 1]  RectangleSizeUnits=m  BrickDimensions=[1 1 1]  BrickDimensionUnits=m  CylinderRadius=R  CylinderRadiusUnits=mm  CylinderLength=L  CylinderLengthUnits=mm  SphereRadius=1  SphereRadiusUnits=m  EllipsoidRadii=[1 1 1]  EllipsoidRadiiUnits=m  ExtrusionCrossSection=[1 1; -1 1; -1 -1; 1 -1]  ExtrusionCrossSectionUnits=m  ExtrusionLength=1  ExtrusionLengthUnits=m  PolygonNumSides=3  PolygonOuterRadius=1  PolygonOuterRadiusUnits=m  ExtGeomFileType=STEP  ExtGeomFileUnits=m  RevolutionCrossSection=[1 1; 1 -1; 2 -1; 2 1]  RevolutionCrossSectionUnits=m  RevolutionExtent=Full  RevolutionAngle=180  RevolutionAngleUnits=deg
  To Ancerstor : PMIOPort  Side=Left
  To Follower : PMIOPort  Port=2  Side=Right
  Reference and Test : PMIOPort  Port=3  Side=Left
  connections:
  Rigid Transform1/RConn1 -- To Ancerstor/RConn1
  Rigid Transform2/RConn1 -- To Follower/RConn1
  Rigid Transform1/LConn1 -- Reference and Test/RConn1 -- Solid/RConn1 -- Rigid Transform2/LConn1

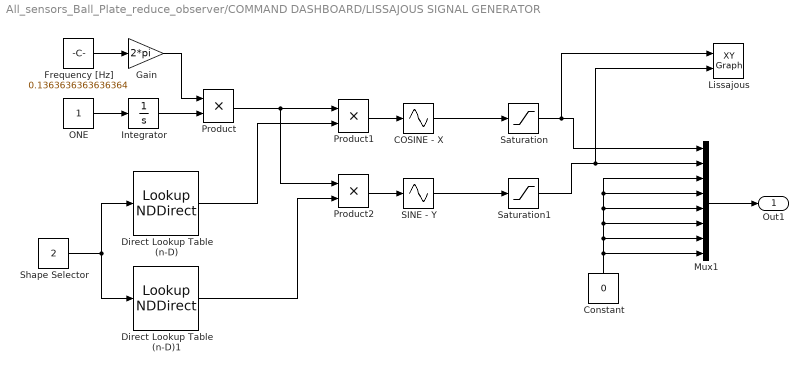
== system All_sensors_Ball_Plate_reduce_observer/COMMAND DASHBOARD/LISSAJOUS SIGNAL GENERATOR ==
  COSINE - X : Sin  TimeSource=Use external signal  Amplitude=0.1957219251336899  Bias=0.03519999999999998  Phase=pi/2  SampleTime=0
  Constant : Constant  Value=0
  Direct Lookup Table (n-D) : LookupNDDirect  NumberOfTableDimensions=1  Table=[0 1 1 3 3 5]'
  Direct Lookup Table (n-D)1 : LookupNDDirect  NumberOfTableDimensions=1  Table=[0 1 2 2 4 4]'
  Frequency [Hz] : Constant  Value=0.1363636363636364
  Gain : Gain  Gain=2*pi
  Integrator : Integrator
  Lissajous : simulink/Sinks/XY Graph  xmin=-1  xmax=1  ymin=-1  ymax=1  st=-1
  Mux1 : Mux  Inputs=8
  ONE : Constant
  Product : Product
  Product1 : Product
  Product2 : Product
  SINE - Y : Sin  TimeSource=Use external signal  Amplitude=0.1830769230769231  Bias=0.064  SampleTime=0
  Saturation : Saturate  UpperLimit=0.2  LowerLimit=-0.2
  Saturation1 : Saturate  UpperLimit=0.2  LowerLimit=-0.2
  Shape Selector : Constant  Value=2
  Out1 : Outport
  wires:
  Shape Selector/1 -> Direct Lookup Table (n-D)1/1, Direct Lookup Table (n-D)/1
  Direct Lookup Table (n-D)/1 -> Product1/2
  COSINE - X/1 -> Saturation/1
  Product1/1 -> COSINE - X/1
  Product2/1 -> SINE - Y/1
  Saturation/1 -> Lissajous/1, Mux1/1
  Frequency [Hz]/1 -> Gain/1
  Integrator/1 -> Product/2
  Gain/1 -> Product/1
  ONE/1 -> Integrator/1
  Product/1 -> Product2/1, Product1/1
  Direct Lookup Table (n-D)1/1 -> Product2/2
  Saturation1/1 -> Lissajous/2, Mux1/2
  SINE - Y/1 -> Saturation1/1
  Mux1/1 -> Out1/1
  Constant/1 -> Mux1/5, Mux1/3, Mux1/4, Mux1/6, Mux1/7, Mux1/8

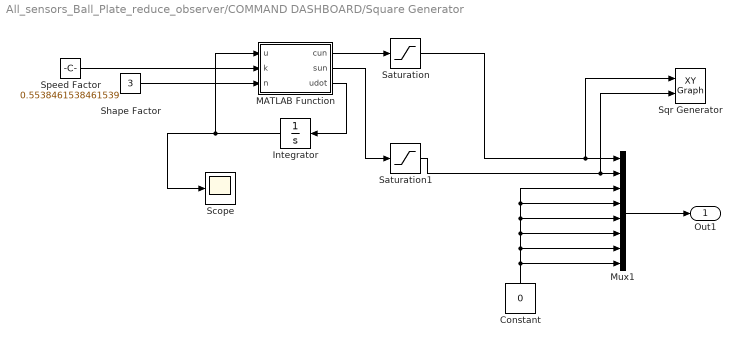
== system All_sensors_Ball_Plate_reduce_observer/COMMAND DASHBOARD/Square Generator ==
  Constant : Constant  Value=0
  Integrator : Integrator
  MATLAB Function : MATLAB Function  TreatAsAtomicUnit=on
  Mux1 : Mux  Inputs=8
  Saturation : Saturate  UpperLimit=0.2  LowerLimit=-0.2
  Saturation1 : Saturate  UpperLimit=0.2  LowerLimit=-0.2
  Scope : Scope
  Shape Factor : Constant  Value=3
  Speed Factor : Constant  Value=0.5538461538461539
  Sqr Generator : simulink/Sinks/XY Graph  xmin=-1  xmax=1  ymin=-1  ymax=1  st=-1
  Out1 : Outport
  wires:
  MATLAB Function/1(cun) -> Saturation/1
  MATLAB Function/2(sun) -> Saturation1/1
  Shape Factor/1 -> MATLAB Function/3(n)
  Constant/1 -> Mux1/5, Mux1/3, Mux1/4, Mux1/6, Mux1/7, Mux1/8
  Saturation/1 -> Sqr Generator/1, Mux1/1
  Mux1/1 -> Out1/1
  Saturation1/1 -> Sqr Generator/2, Mux1/2
  Integrator/1 -> MATLAB Function/1(u), Scope/1
  MATLAB Function/3(udot) -> Integrator/1
  Speed Factor/1 -> MATLAB Function/2(k)

== matlab function All_sensors_Ball_Plate_reduce_observer/COMMAND DASHBOARD/Square Generator/MATLAB Function ==
  data: u input; cun output; k input; n input; sun output; udot output
function [cun, sun, udot] = fcn(u, k, n)
%#codegen

%y = k/(0.001+((cos(u)^2*sin(u)^(2/n - 2))/n^2 + (cos(u)^(2/n - 2)*sin(u)^2)/n^2)^(1/2));
NUM = sin(u)^2 * cos(u)^2;
DEN = sin(u)^4 * (cos(u)^2)^(1/n) + cos(u)^4 * (sin(u)^2)^(1/n); 

cun = 0.15*sign(cos(u))*power(abs(cos(u)), 1/n);
sun = 0.15*sign(sin(u))*power(abs(sin(u)), 1/n); 
udot = k * n * ( (0.001+NUM) / (0.001+DEN) )^(1/2);
